simulink model "simulinkArduinoNN"  (R2020b)
settings: Solver=ode3  StartTime=0.0  StopTime=inf  FixedStep=0.05  RelTol=1e-3
libraries: neural x6, arduinolib x3, simulink x1
(part 1 of 2)
settings Model: FPTRunName=Active  SILPILModeSetting=veronly  ExtModeTrigDuration=2  Creator=The MathWorks, Inc.  LastModifiedBy=anton
settings DataIOCC: LimitDataPoints=on  SaveFormat=Array  ReturnWorkspaceOutputs=off
settings OptimizationCC: ExpressionDepthLimit=2147483647  LifeSpan=Inf  MaxStackSize=64
settings DebuggingCC: UnderspecifiedInitializationDetection=Classic  MergeDetectMultiDrivingBlocksExec=none  FcnCallInpInsideContextMsg=warning  AllowSymbolicDim=off  StateNameClashWarn=warning  SFUnexpectedBacktrackingDiag=warning  SFNoUnconditionalDefaultTransitionDiag=warning  SFExecutionAtInitializationDiag=none  ArithmeticOperatorsInVariantConditions=warning
settings HardwareCC: ProdBitPerInt=16  ProdBitPerPointer=16  ProdBitPerSizeT=16  ProdBitPerPtrDiffT=16  ProdLargestAtomicFloat=None  ProdWordSize=8  ProdHWDeviceType=Atmel->AVR
settings ModelReferenceCC: PropagateSignalLabelsOutOfModel=off
settings SFSimCC: SimUseLocalCustomCode=off  MATLABDynamicMemAlloc=off
settings RTWCC: Description=Embedded Coder  SystemTargetFile=ert.tlc  HardwareBoard=Arduino Uno  TemplateMakefile=ert_default_tmf  GenerateReport=on  RTWVerbose=off  RTWUseLocalCustomCode=off  Toolchain=Arduino AVR  BuildConfiguration=Faster Runs  LaunchReport=on
settings CodeAppCC: ForceParamTrailComments=on  OperatorAnnotations=on  StateflowObjectComments=on  MATLABSourceComments=on
settings ERTTargetCC: MultiwordLength=2048  ERTCustomFileBanners=off  SupportContinuousTime=on  SupportNonInlinedSFcns=on  RemoveResetFunc=off  SupportVariableSizeSignals=on  ModelStepFunctionPrototypeControlCompliant=off  ExtModeStaticAllocSize=250
settings ConfigComp: CovMetricSettings=dw  CovSaveCumulativeToWorkspaceVar=on  CovSaveSingleToWorkspaceVar=on  CovExternalEMLEnable=off  CovSFcnEnable=off

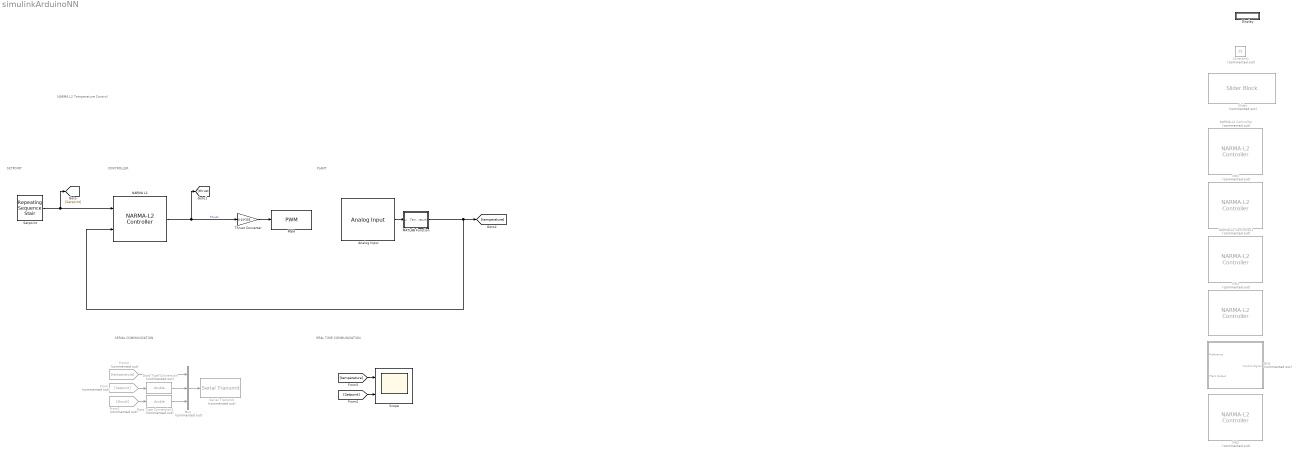
== system simulinkArduinoNN ==
  note: PLANT
  note: NARMA L2 Temperature Control
  note: CONTROLLER
  note: SETPOINT
  note: SERIAL COMMUNICATION
  note: REAL TIME COMMUNICATION
  Analog Input : arduinolib/Analog Input  pinNumber=0  ReadResultsOnly=off  ConversionTriggerSource=Software  ExternalTriggerType=uint32( 0 )  OutputDataType=uint16  EnableConversionCompleteNotify=off  EnableOuputStatus=off  SampleTime=0.05  blockPlatform=arduino
  Constant1 : Constant  Commented=on  Value=25
  Data Type Conversion : DataTypeConversion  Commented=on  OutDataTypeStr=double
  Data Type Conversion1 : DataTypeConversion  Commented=on  OutDataTypeStr=double
  Display : Display
  From : From  Commented=on  GotoTag=Setpoint
  From1 : From  Commented=on  GotoTag=thrust
  From2 : From  Commented=on  GotoTag=temperature
  MATLAB Function : MATLAB Function  TreatAsAtomicUnit=on  SystemSampleTime=0.05
  Mux : Mux  Commented=on  Inputs=3
  NARMA L2 : neural/Control Systems/NARMA-L2 Controller  Normalize=0  IW1_1=[0.040017528221302098301 0.038720566252876224833 0.00064587793429901456128;-0.34244510037897918364 -0.83577023563736208001 -0.98984885365635955079]  IW3_2=[1.7482699976429136868 1.6815146793184658769 1.4643769373344286411;0.19971534547986175001 -0.23761110741996102624 -0.8313049704497363912]  IW5_3=-0.034754252519757541928  LW2_1=[2.5400144996497338035 -0.95992293938881778637]  LW4_3=[0.40171315691149905858 1.6229597477464516864]  LW5_4=-0.69241708190501793929  LW6_5=0.30729820790646955597  LW6_2=5.1056684069757363176  B1=[-2.0653006877227757521;12.38881103090871072]  B2=4.1767028794970464389  B3=[11.273095141969324828;-4.8446886512396289959]  B4=0.11110386902302692158  Limit_output=0  min_output=0  max_output=0  Use_Previous_Weights=1  Ts=0.05  S1=2  Ni=2  Nj=2  sim_file=0  trainfun=trainlm  Use_validation=1  Use_Testing=1  max_i=100  min_i=0  max_i_int=0  min_i_int=0  sam_training=0  epochs=200  minp=27  maxp=89  mint=20.399999999999998579  maxt=89
      settings: SourceProductBaseCode=NN
  NARMA-L2 Controller : neural/Control Systems/NARMA-L2 Controller  Commented=on  Normalize=0  IW1_1=[-0.41816835291281462261 -0.35264418343474912554 -0.32086643568429712436 -0.32416679636657497188 -0.2456158726033293993 -0.20850521425442761214 -0.18289108034733025931 -0.21218563723547304023 -0.21419207008282342697;2.5549495009601193019 2.6646789452516004282 2.5419717505159939996 2.6551200807204047294 2.6409125333066105767 -0.21625379401632879861 -0.13882591817244868682 -0.18729539371465481201 -0.2168326394422463721;-1.2721943805663364913 -1.4939241912413336877 -1.4732825136080858197 -1.3301923784215392565 -1.3766079352876294806 -0.21157536269805202189 -0.35794012087187238036 -0.2715608750426205531 -0.099217006228763698905;4.7245056370737605889 4.8750083803908825786 4.8406385609924518221 4.7287810787814468227 4.9015338893010964583 2.9977258587230961595 2.9962052565501506862 2.9831973505122002521 2.9895567642981588641;0.0082199585455147387153 0.0064845805330013064904 0.006075874243255548722 0.0067791387839133522911 0.0061881761888035770325 3.7344261662485848041e-05 -2.574807479513796659e-05 -7.8717489178539200106e-05 8.9401831986167490488e-06;0.15145529963067391743 0.081246220641696509368 0.09126813427485024055 0.020684568354657238004 -0.024788994416876992954 0.020484030560411779776 0.024664224602330322988 0.038649647286030541782 0.053796682116574512378]  IW3_2=[0.14756453407069930472 0.038071892914692956333 -0.29594778362426327201 -0.069820362182882428348 0.70962571362936266439 -0.039960254460013666655 0.014433276009520068853 -0.03849288617468893392 -0.0063373593751587260076;-0.037939280094850681702 0.19900877381833009805 -0.38798657450907908517 0.25323889327365478596 -0.22696331218004994756 -0.022003323386020349345 -0.25009301164211789059 -0.073915899763233594566 -0.0031735084905345602516;-0.13125875378245754899 1.5478009170062148048 -0.16796755957035469642 -0.24328743276964936992 0.78159866568757363492 -0.087276474157856082092 -0.79951436698558953076 -0.18032038380962273072 0.50260101455877292942;-0.98396806059596020333 1.8995275827316164818 -2.1897842904461501945 -2.2973087662015334587 0.74482251566342538851 0.37391416368970209483 -0.26168694683679905033 0.52694681588132086247 -0.20081389809051350404;-0.84654678308830177969 0.23674069355138971371 -0.85750959855860364733 -0.0029026755591129841695 0.80240107648048308864 -0.26949776994017687892 0.58963130621671644427 0.060296956437784550442 0.025326443244529463217;-1.0595645910632840447 -2.2049697211214853709 -2.5865975981986322196 -1.4166077816243936027 -0.42474198506086918714 1.0053275099646519219 -0.1646434860624376717 1.1625718032264895641 -0.042783101732736306122]  IW5_3=-0.50023824145104556216  LW2_1=[-0.079625603267581251954 -1.3542538026665085216 1.527768373182599948 -0.1693983456685116129 -4.2945392435147784482 -0.66985082816128915795]  LW4_3=[-0.23005208282157874056 1.1169727507123785593 5.2260595457114993323 0.15271392956959686793 3.227767721365951914 0.53482218884047061369]  LW5_4=-0.31498488126420315369  LW6_5=0.00011717498325399218278  LW6_2=-6.8954901337929515037  B1=[5.4002255193728867511;-5.0577886183983151724;1.840287386760475874;-3.0763976357700304476;-0.94496016942633787039;1.4506208908622164611]  B2=-0.4300654600706715347  B3=[0.98059537611604463692;-1.6514227306205062629;2.0674947612374428019;-4.0204934657747450899;-0.13870728866110765276;-5.1640535704469163747]  B4=0.0042934946030275117357  Limit_output=0  min_output=-Inf  max_output=Inf  Use_Previous_Weights=1  Ts=0.2  S1=6  Ni=5  Nj=5  sim_file=ball  trainfun=trainlm  Use_validation=1  Use_Testing=1  max_i=100  min_i=0  max_i_int=0.2  min_i_int=0.1  sam_training=100  epochs=100  minp=0  maxp=93  mint=21.399999999999998579  maxt=93
      settings: SourceProductBaseCode=NN
  NARMA-L2 Controller1 : neural/Control Systems/NARMA-L2 Controller  Commented=on  Normalize=0  IW1_1=[0.021297476685584439127 0.020671547447015964361 3.6994772399302055111e-05;0.20573585021771889636 0.23002083189625410764 0.22530022103732963434]  IW3_2=[-0.46310314388711848466 -0.18941619784751775879 -0.07042384218363256787;0.59986875760900981724 0.42193527769695915453 -0.027483551883907161167]  IW5_3=0.5633369451363166025  LW2_1=[-4.3800886706593535891 -1.907929921162713649]  LW4_3=[0.4170003926895888835 1.4758854178100675458]  LW5_4=0.54195412905265116787  LW6_5=-0.001961000929507238609  LW6_2=-5.4691828879464159385  B1=[-1.0898449945740975586;-6.7681089120354176458]  B2=-2.8436322564684024528  B3=[9.4686029787908267963;-3.2224033771547984095]  B4=0.99133763358280613254  Limit_output=0  min_output=0  max_output=0  Use_Previous_Weights=1  Ts=0.05  S1=2  Ni=2  Nj=2  sim_file=0  trainfun=trainlm  Use_validation=1  Use_Testing=1  max_i=100  min_i=0  max_i_int=0  min_i_int=0  sam_training=0  epochs=200  minp=27  maxp=89  mint=20.399999999999998579  maxt=89
      settings: SourceProductBaseCode=NN
  NN1 : Subsystem  Commented=on  AncestorBlock=neural/Control Systems/NARMA-L2 Controller  mask(NARMA-L2 Controller){Normalize=0, IW1_1=[0.081001796331336056722 0.15736369236145394956 -0.0061189171765253010798 0.031259373269709643528 -0.29161810270363336395 0.038960711989141236233 0.21066716241391639231 0.33564336592970134276 -0.42429187654869637836 -0.10771109383123129988 0.30271654934038322304 0.25669185229126045833 -0.18814574524270602507 -0.70360581796463639304 0.0022722054824509882454 0.22910624679545782412 0.31712007292734828434 -0.089593213208105274004 -0.29265065772660509014 0.25268525353674159417 0.40327134398474917543 0.10002475107419414591 0.10633957135057141297 0.22378520139222193852 -0.035441999466167897759 -0.09543965847989055451 -0.078475621102576539889 0.7978101624930962199 0.79197484966292575059 -0.75869567511731361709 -0.53133263705840783064 -0.40463183765462173991 1.4449740542986064806 1.423356606533091373 0.71567488745926521876 -0.71695273665588032941 -2.4976194364111630186 -0.52233538556271086328 -0.25784969469923535446 0.32001986891446365657 -0.34199391648141252986 0.21622613985873931353 0.51601933874237093658 -0.10229354784308368476 -0.063445068067935039835 0.76782685785385373922 0.58773337673444869811 -0.21322284745124506222 -1.3054574307789652554;-0.45565673055947875092 -2.8918895554005401571 -0.55732675097013917309 0.41047627061890573641 -1.0670853854999666765 -1.2269041735405823434 -0.53267398056508041826 -0.97207552132808006107 -1.5722657868604021925 -0.53941889635209872012 -0.032041342375024699229 0.09039551516666352593 -0.24629516613116916868 0.11927248975686825794 -1.2163427500639183432 0.94175325425605316276 -0.61664065600630824093 1.2537434811038190574 1.9708242434192153603 -0.18910074831646658811 1.1517160053052737378 -0.20615377037471419031 0.70037457310627138085 0.17251062422370158633 0.053382827490675487103 -1.651565422525036686 1.6906721755139886287 1.1022326413130534295 0.62515064205556036825 1.1201224089032946196 1.2824320188391788999 1.1251907270244796422 0.975294135970491749 1.2712381874161382544 1.8243027831043623355 -2.0127819149324448489 -1.9988806349665289019 0.0060280342477723233147 -0.028997473490317924455 4.2722776160136408663 0.96387017843053901522 -0.43562173505830670273 -1.0910256304234176028 -3.077903779867181111 -0.62300090522248086078 0.59335314064570743309 -0.10375978052824513798 -0.6895512783715659344 0.095697058256527731124;-0.042425975032530191533 -0.020290500259480211132 0.0020558665614247998224 -0.016851639980462271989 -9.5877759916884074858e-05 -0.00043919734009329294052 -0.02432381886257231618 -0.017583525777367700615 -0.017441386778719040335 -0.0040392297673593619001 -0.0038313554643087392899 0.0070579402620235629634 0.0078744850566811568082 -0.013939382367620677117 -0.0069330983391031903579 0.006428303090721439704 0.0076925694344603182118 -0.010213041618125990456 0.015297975743313978192 0.0069861958830649481533 -0.00039084881779854097235 -0.008621454336059724069 0.011403063240721680177 -0.027621446781558738753 0.0024782386744561469769 -0.0013077434278823262415 -0.00010498714836182009241 -0.0011898238650083332001 0.002668977180136910491 -0.00074960605879568792832 -0.0066212455474144917694 0.0036782537344367594902 0.0024779959822594154958 -0.0007716761197923681934 0.0060692515023587755713 -0.010470727481629332756 0.00651595757366603065 -0.0044179300248572807644 0.0023095130361779712264 0.0032279872975385253721 -0.0019027991455841971984 0.0030634915133303550032 -0.0039399868098482868778 -0.00029080766799168656462 0.0025879809946031118173 -0.00089996436815702825131 -0.0027431045461358116028 0.0015161575681175442926 0.00055000124936672957141;0.13973537349263717711 -0.030466654127967104926 0.13187207328935218742 0.08049426006455617788 -0.076243603851158442408 -0.16547014579527388745 -0.043008846385773881471 -0.11950007788257802077 -0.046614671001138807682 0.16047901716290213781 0.073120480998826051233 0.093856529495385407347 -0.24557469126930167591 -0.19531757450559239508 -0.25070881757410712343 -0.31477274386096759651 -0.23489476856896024382 -0.029056344281550659098 0.035279823771276613842 ...(+19340 chars)], IW3_2=[0.28221035721372655924 0.24949048164687237517 0.50091503695658035067 0.29138375416878581348 0.3047008394534790332 0.3601462353909597458 0.40525095161513946529 0.26607434365595128423 0.55636218982740370809 0.34241447621358733766 0.36922712946264368838 0.45012806085967455028 0.39746229989535664107 0.3517864672941124482 0.4414843841493564236 0.36597247241314873056 0.35722161160362497778 0.44166531166398254049 0.16265027540472642986 0.25024861114207264112 0.30989912765920363258 0.41245163179350691207 0.33932632574725996033 0.49564568667022140813 0.57942154725730332654 -0.41461285525358454462 -1.2532697594117170325 -1.016361035663570167 -0.50321252693688756086 -0.54111297537343439057 -0.64187004471658015703 -0.14877502282026722202 0.60233695514965923667 1.0051459831346829521 0.94121331461014512421 1.2528330966171683514 1.2616527525012983801 1.2522219802105709618 1.2306525532073226969 1.2285383897761898986 1.2223848740139509061 1.3599109870888566043 1.4151603107720585051 -0.24410711433607779064 -0.2618941587969862983 -0.29246174834972238354 -0.30083689664157564625 -0.3068812201344749413 -0.28850938424857819342;1.0039073009269712244 0.55909515429426293043 0.35983620274181782328 0.070909546265178188817 -0.31883710307836060638 0.021145812343666886557 -0.14052154577085901321 -0.3271388918228536058 -0.3056633047260269298 -0.1623172750176906376 0.27797165474081836356 0.15225869328795568758 0.07363456490444941771 -0.62576865843504525522 -0.049087382425018186161 -0.30920133067014099471 0.076637081473032608869 0.14304981128415980574 -0.036499429525520703244 -0.2347509035584434689 -0.26179516887628079269 0.31296574936306986725 -0.15475190365927896097 0.35308581539443995023 -0.10202609695406412993 -0.17396380085010321181 0.096710134721432985949 -0.20830070808662115578 -0.47058670424406728872 0.52295605161493230462 0.0094320573624777082067 0.06715455531127276223 0.04187265104715939823 0.30327034992914059242 0.20145747764813776159 2.0909735274704814856 0.84704439041569612456 0.50997408572182101327 0.30641972313442999987 0.19197087648156632711 -0.60791406184183405248 -0.59405380909595950634 -0.034990495138219557258 -0.069266505872329714455 0.21048086131964355294 0.22667210136932716691 0.042230258564031453172 0.03593561616959382865 0.053541505760580782036;-1.2112673056771381397 1.3552795429509238989 0.001340057277427330858 0.78347666775327995392 1.822361998970581709 0.5122989014137333541 -0.50111071047377020449 1.0617013213073929201 0.58128441457677981763 0.54344476225833260319 0.1944925038947179774 -0.43659907148292809165 1.707053424524483054 2.3777386093428747316 1.0594342712117987837 -0.35201497834900069561 -0.26906184398102572786 0.42788289669276663441 -1.4076861875310526795 0.19171855087256500783 -0.16925887294509342484 0.71966576151787531312 0.72059248245890283879 0.40053926618387347691 1.1464662234770182092 0.21463009737624402784 -0.80154327712810713447 -1.0629457174136294206 -1.0210941619912747846 -2.2004122602064311032 -1.9521985738729117354 -1.7172947022930669103 0.97621035059419447588 -0.44761702689860249915 0.77989707551171627564 0.40531267147789640237 1.1532982191938567773 1.1091066563735785255 1.4501837944712221429 1.6347891876696920566 1.3043885869211773176 1.4130197077664012895 0.91046411495307311146 -2.574445641552231212 -2.2214038450268880354 -2.6731230845813365171 -2.0029579616587414037 2.3026763340089528853 0.10442858352341162498;0.49547962694450214949 0.4634582007650282498 1.0890686566832370463 0.55177896616662225338 0.42636275537373924394 0.50771505829480712002 -0.12407657734639600255 0.32044081185938477763 0.81178540200128224136 0.43724654422399117371 -0.062071306632406897386 0.17905919149878501972 0.32630694572714147306 1.2520944876042674476 0.57891801858243330248 0.50502835376602539519 0.44893767424576869196 0.98344432483845856119 0.75591969357376931349 0.5511071553167703474 0.76629856245022498484 0.062215397882230967508 -0.15232706678745877582 -0.057308435995030514165 0.050820622281957550381 2.013762225413406437 ...(+18729 chars)], IW5_3=0.049794786120951804731, LW2_1=[0.019522040564175939525 0.010030780829141647259 -2.9269869808931687771 -0.044720248183330521541 3.3896735937268989147 0.055333660288906100222 -0.046769359291137894974 0.72657606414846986898 -0.231739559939226486 -2.8734140238129448619 -0.72738980090921023791 -3.1703753625289112783 0.030516532724820310402 -0.011164868475765466621 -2.6504898493220547806 -0.017243119800886514553 -3.6192209431664785768 0.062752740912268317741 -3.4737778709395779053 -0.020630211384971723632], LW4_3=[-0.49767595711144158033 -5.0418393908440179985 3.5744239145482166187 -3.9384524981309438907 -4.8073499402252970469 2.727310872235649164 -0.71730478292060606549 0.12740639700024902758 -4.6201956999409405924 4.0234022300950194051 5.8975918809235290396 1.9099313228049630276 0.22431709645351263771 4.1350604422295358376 3.8128713144263901569 5.2889865099553734495 5.1501748174827808313 -2.0783275816180553086 0.87022382331586878301 5.2226018567932683823], LW5_4=0.25213902069175248011, LW6_5=-0.0018683962758275409616, LW6_2=1.0196993926720294699, B1=[-13.683970472853349776;-10.829168374571350952;3.2499778850305398592;12.860073554387984274;-4.3007772967563742128;-12.715349009048415141;6.4787516301547949382;-19.564844579552055137;0.20783599937462277074;-5.7023611773114426526;10.113035508787838523;13.286447344365756251;2.8802714807787950235;26.296794390935232855;-0.69066711291984395071;-0.52575739785160779949;-8.8606049427338184898;-14.753008137324961524;1.7681866839940678648;10.252069531512537637], B2=3.7097017031416461563, B3=[0.15043469453056407259;2.9756978074974016479;7.1920582605238250196;-9.8267085343876328096;-1.1888977589751141828;-10.309826346565044375;-5.3298483838539478796;6.2524100723987032779;-3.1661464323339654214;-10.512300523957687659;-10.477978044887745313;-9.6945816023752779955;-15.116599806060138533;11.336838798593424471;11.996325424358646572;-0.47776234751081703145;6.2912996815758619462;2.9850645554334387377;2.5315214878778347085;19.896605647385079862], B4=2.3815464859015680332, Limit_output=0, min_output=0, max_output=0, Use_Previous_Weights=1, Ts=0.05, S1=20, Ni=25, Nj=25, sim_file=0, trainfun=trainlm, Use_validation=1, Use_Testing=1, max_i=100, min_i=0, max_i_int=0, min_i_int=0, sam_training=0, epochs=100, minp=4, maxp=94, mint=20.899999999999998579, maxt=94}
      mask prompts: Ts "Sample time"; trainfun "Training function"
      mask help: NARMA-L2 Controller. You first train a neural network model of the plant to be controlled. The controller is a rearrangement of the trained plant model. Double-click the NARMA-L2 Controller block to begin the plant training.
      mask init:
      | network;
      | x1 = [0    .4   NaN  .33  .55   .55  .33  .33  NaN .80  .92 .92];
      | y1 = [.95 .95 NaN  .75  .75   .55  .55  .75  NaN  .95 .95 .65];
      | x2 = [0    .43 NaN .45 .45    NaN .92 1.2 NaN .63 .85 .85 .63 .63 ];
      | y2 = [.39 .39 NaN  .41 .55   NaN .65 .65 NaN .75 .75  .55  .55  .75];
      | x3 = [.45 .45 NaN .42 .45 .48  NaN .33 .4 .33];
      | y3 = [.75 .90 NaN .83 .90 .83  NaN  .98 .95 .92];
      | x4 = [.75 .75 NaN .72 .75 .78  NaN  .5 .7 NaN .63 .7 .63];
      | y4 = [.75 .90 NaN .83 .90 .83  NaN .95 .95 NaN .98 .95 .92];
      | x5 = [.43 .43 .77 .77 .43 NaN .36 .43 .36 NaN .75 .75];
      | y5 = [.37 .41 .41 .37 .37 NaN .42 .39 .36 NaN .41 .55];
      | x6 = [.92 .92 .77 NaN .84 .77 .84];
      | y6 = [.65 .39 .39 NaN .42 .39 .36];
      | x1t=.03; y1t=.31;
      | x2t=.03; y2t=.85;
      | x8t=.03;y8t=.21;
      | x3t=.77; y3t=.53;
      | x4t=.77; y4t=.44;
      | x5t=.34; y5t=.49;
      | x6t=.58; y6t=.49;
      | 
      | 
      | t=(0:24)/24*2*pi;
      | xs = .05*cos(t);
      | ys = .05*sin(t);
      | xs1=xs+.45;
      | ys1=ys+.95;
      | xs2=xs+.75;
      | ys2=ys+.95;
      settings: OpenFcn=nncontrolutil('nnident','',gcbh,gcb,'narma_l2');
      mask Help: helpview('deeplearning','nnet_narma_l2_controller');
      mask TypeOptions trainfun: trainbfg | trainbr  | traincgb | traincgf | traincgp | traingd | traingdm | traingda | traingdx | trainlm  | trainoss | trainrp  | trainscg
      mask Display:
      | e = 0.06;
      | c1 = [120 150 230]/255;
      | c2 = ([120 150 230]+0)/383;
      | c3 = ([120 150 230]+128)/383;
      | patch([0 1 1 0],[0 0 1 1],c1);
      | patch([0 1 1 1-e 1-e 0+e],[0 0 1 1-e 0+e 0+e],c2);
      | patch([0 0 1 1-e 0+e 0+e],[0 1 1 1-e 1-e 0+e],c3);
      | plot([[x1 NaN x2]*.9-.075 ], [[y1  NaN y2]*.9-.1 ]);
      | plot([[x3 NaN xs1 NaN xs2]*.9-.075 ], [[y3 NaN ys1 NaN ys2]*.9-.1 ]);
      | plot([x4 NaN x5]*.9-.075,[y4 NaN y5]*.9-.1);
      | plot([x6 NaN ]*.9-.075,[y6 NaN ]*.9-.1);
      | plot([0 1 1 0 0],[0 0 1 1 0]);
      | text(x1t,y1t,'Plant');
      | text(x8t,y8t,'Output');
      | text(x2t,y2t,'Reference');
      | text(x3t,y3t,'Control');
      | text(x4t,y4t,'Signal');
      | text(x5t,y5t,'f');
      | text(x6t,y6t,'g');
  NN2 : neural/Control Systems/NARMA-L2 Controller  Commented=on  Normalize=0  IW1_1=[0.42999578451454106842 0.20519526356674350209 0.48560842768546641501 0.45796392885806858075 0.56450148087544238518 0.50351630398968461044 0.40693748816290253867 0.42403535086980548297 -0.58936365396049317233 -0.30903885679007220277 -0.22292526287955208297;0.25841032509566608244 -0.13737805067406735904 -0.15482151715535916181 0.65297703160385611731 0.17274411066130934689 0.40453996700577132817 -0.4111114686333410817 0.36147208605498298839 0.021131113938576966127 -0.14014771021062302769 0.092839271051875879581;-0.011434700121978670986 -0.010720729619677252242 -0.0096564374143097118919 -0.0082604891885513388045 -0.0096005768011547358565 -0.010391114612203487463 -1.0476759531353016286e-05 7.2077522336085755677e-05 -9.6420386119362220373e-05 8.2917824210678723652e-06 2.3416884195674133776e-05;-0.56744746474663465552 -0.47940353954936382186 -0.36673868830426242793 -0.72388284193056895433 -0.22890654036687180239 -0.62816667955451999106 -0.15556880492137584171 -0.27089640898497230337 -0.1535093393110727733 -0.72590483691104790154 -0.80082100631588459816;0.63814745459816246687 0.6401406546649579532 0.26654247833268734924 0.2952640512926372196 0.84955032500919014371 0.21317123129875506504 -0.29465041983107009838 -0.19037508756029189461 0.15397062431184516118 -0.07918764571200906377 -0.049066929249987248363;0.68031528203635949215 0.37921354169754795116 -0.022222469467425922524 2.0972653722608960436 0.40664857275118748703 1.4365602546419606877 0.16120398009003295003 0.033632347331193010453 -0.20163202670797347738 -0.58984661369907187556 -0.91883922634755954562]  IW3_2=[0.62072958787989240825 0.48642642668883517842 0.8143032356552284412 1.1295518407252980175 -0.12252819519746503685 1.3035863364893975902 -0.061540668235754963922 0.13396836381379054193 -0.97273489523940537271 -0.57449054628195250771 -0.79552860018882165516;0.022148742001209309471 0.35509226217601974618 0.15936552561537462025 0.41743348717457334773 0.21671159251167160242 0.21588238211386889809 0.10365014565444288785 0.32399157654972332576 -0.24370824872351357082 0.1052740296345326676 0.21533119379063728194;-0.34960873325137170609 0.60597565806765596452 1.122135647654741053 -0.20643521097916414653 0.71677006726172487472 0.30105254139888160125 -0.12032940047543728979 -0.37497085528307366742 0.34043889151749706645 -0.36823126955913926261 -0.11653268522074718139;0.19393773260013844051 0.067610881920749932306 0.23399090778869918728 0.21457707930399366747 -0.14374410046381749795 0.26692484357754975299 -0.17370341744012737784 -0.06060480970759270225 0.25309705955902561669 0.086487428730836077295 -0.042775161104023948222;0.97957315902225849946 1.1975315558082157974 0.94192073634989559316 1.2208743757048998724 1.3045447227043793781 1.0252258514225500718 0.17267256498501859507 -0.27917778045509750173 -0.21332665529313060704 -0.94663326100635658555 -1.4586763385411685157;-0.13919708229624574991 -0.04346517225565629805 -0.26370853710094882549 0.28690607977414084306 -0.38642813425088834434 -0.033589343275048713644 -0.02182821320742767135 0.0546643245090925739 -0.093743190688845248748 -0.083182309228358813913 -0.23796081789112336069]  IW5_3=0.00035625599399004379431  LW2_1=[0.0097832663468938908802 -1.6727188551373248782 4.0745823001807295327 0.70095287853249088617 -1.5696668938645457203 -0.0037480653401194630528]  LW4_3=[-1.3975705228945904945 0.5017185102204857472 2.1171483657331444661 -0.28696914872047785128 -0.97527522346300143941 0.42327247399147505114]  LW5_4=0.30108920563813407201  LW6_5=-0.64763974290970649506  LW6_2=-4.0888519730117227624  B1=[-12.820258601526894893;8.3658161662943157921;1.4697304281208545262;2.3120851336475483073;-3.5099662930913710923;-7.2883678124612831795]  B2=-2.0492682323172446424  B3=[-12.875713784252596383;-2.8354269756645469336;-6.0083619963053065405;-3.7653708851426892501;5.4665583507364479132;7.3625549242107526382]  B4=-0.58721073754749031348  Limit_output=0  min_output=0  max_output=0  Use_Previous_Weights=1  Ts=0.05  S1=6  Ni=6  Nj=6  sim_file=0  trainfun=trainlm  Use_validation=1  Use_Testing=1  max_i=100  min_i=15  max_i_int=0  min_i_int=0  sam_training=0  epochs=200  minp=18  maxp=98  mint=21.600000000000001421  maxt=98
      settings: SourceProductBaseCode=NN
  NN3 : neural/Control Systems/NARMA-L2 Controller  Commented=on  Normalize=0  IW1_1=[-1.8593597747394099429 -1.7868866101544693681 -1.8040454788392301655 -1.9838257421676190884 -0.59666751207188750694 -0.36769528636219883655 -0.34025561862194281249;0.2407352589535642351 0.0050481122489959336791 0.16276896799883461275 -0.035062703388723560904 -1.9821712665394159991 0.31150538924206866431 0.78895516926670472557;-1.0553795633231950468 -0.57149741310900725733 -0.63698486339372162313 -0.84567298056237627524 0.26193724484567859623 0.088310780559837709358 0.14623445800203638267;0.066739972037093212021 0.065640937616500610874 0.065153243927194043339 0.063409055986086829138 0.16345948581467512062 0.0027269730479867575201 -0.1648645583778025614]  IW3_2=[1.7046755888591129668 -0.55977346676490491451 0.72201571534367703364 1.2642210316096404998 -0.44079893346189036318 -0.72904413580500726511 -0.6362067809622451442;1.0620484567858403668 -1.3485199926093252021 0.49000694606092393135 -0.015393135662842690956 -0.16849501083911408439 0.38667110920263531026 0.16256681105137527066;-0.7012561439499146454 1.7385213775647028189 0.21074420677733413099 0.95396680803443389962 -0.14964373515834350492 -0.38537693641681164403 -0.085595421593214204847;1.0377517806041176573 0.84928740600458496601 0.90102978831172819696 1.1271033981427427406 0.24097268421339421152 -0.75447803864772344795 -0.48909531887179147347]  IW5_3=-0.16390541259389582174  LW2_1=[-1.4762524845472095869 0.63087060840783315552 -4.2448837120043592108 1.5275490537290852266]  LW4_3=[0.79100046595674211591 0.85781251730787477783 0.048117009625120721328 -0.6772590013087830263]  LW5_4=-0.41174696061974336292  LW6_5=0.015996614518592806864  LW6_2=3.0314136397104647358  B1=[1.6639896443073554089;11.553670577041316392;-6.6682157263927992474;-6.7903449650803366922]  B2=3.4671841392617350763  B3=[-8.121899443586778844;-9.400278654001951395;5.7304241453194100231;-7.3885913858366718543]  B4=-0.94276067192527990279  Limit_output=0  min_output=0  max_output=0  Use_Previous_Weights=1  Ts=0.05  S1=4  Ni=4  Nj=4  sim_file=0  trainfun=trainlm  Use_validation=1  Use_Testing=1  max_i=100  min_i=0  max_i_int=0  min_i_int=0  sam_training=0  epochs=200  minp=27  maxp=89  mint=20.399999999999998579  maxt=89
      settings: SourceProductBaseCode=NN
  NN4 : neural/Control Systems/NARMA-L2 Controller  Commented=on  Normalize=0  IW1_1=[0.033013126437020305637 0.085013792551483613469 0.18514597983222294553;-0.012410318240880641866 -0.011382691894752767006 6.5738215801172246943e-05]  IW3_2=[0.083091120238041507595 0.11103244018490328326 0.17835362231576715186;-0.16650598233140753712 -0.092983616630965118532 -0.1864385304900478546]  IW5_3=0.046639341500695291609  LW2_1=[2.3859988149813977643 -6.1735505599395903431]  LW4_3=[0.34565448381951746626 -0.2586640207729006824]  LW5_4=0.49357738618229340943  LW6_5=0.066890877451304661672  LW6_2=6.8012134303038482841  B1=[8.2006268849016628053;0.66737725498513145173]  B2=1.7444785303968004531  B3=[1.9940303734914290867;-0.29693530891239544589]  B4=0.54968670379825324002  Limit_output=0  min_output=0  max_output=0  Use_Previous_Weights=1  Ts=0.2  S1=2  Ni=2  Nj=2  sim_file=0  trainfun=trainlm  Use_validation=1  Use_Testing=1  max_i=100  min_i=0  max_i_int=0  min_i_int=0  sam_training=0  epochs=100  minp=0  maxp=93  mint=21.399999999999998579  maxt=93
      settings: SourceProductBaseCode=NN
  PWM : arduinolib/PWM  pinNumber=6  frequencyType=Default  desiredFrequency=490.2  achievableFrequency=490.2
  Scope : Scope  NumInputPorts=2
  Serial Transmit : arduinolib/Serial Transmit  Commented=on  portNumber=0  sendmode=println  sendformat=Decimal  floatprecision=2  blockPlatform=arduino
  Setpoint : simulink/Sources/Repeating Sequence Stair  OutValues=[24 28 32 28 24].'  tsamp=310  OutMin=[]  OutMax=[]  OutDataTypeStr=double  OutputDataTypeScalingMode=double  OutDataType=fixdt(0,8)  ConRadixGroup=Best Precision: Vector-wise  OutScaling=2^-12
  Slider : SliderBlock  Commented=on  ScaleMax=255
  Thrust Converter : Gain  Gain=0.01*255
  wires:
  Analog Input/1 -> MATLAB Function/1(u)
  MATLAB Function/1(Temperature) -> [temperature], NARMA L2/2
  Data Type Conversion/1 -> Mux/2
  Mux/1 -> Serial Transmit/1
  Thrust Converter/1 -> PWM/1
  NARMA L2/1 -> [thrust], Thrust Converter/1  "Thrust"
  Setpoint/1 -> [Setpoint], NARMA L2/1
  Data Type Conversion1/1 -> Mux/3
  From/1 -> Data Type Conversion/1
  From1/1 -> Data Type Conversion1/1
  From2/1 -> Mux/1
  [temperature] -> Scope/1
  [Setpoint] -> Scope/2
